simulink model "geometric_control"  (R2023b)
settings: Solver=VariableStepAuto  StartTime=0.0  StopTime=20.0  RelTol=1e-3
InitFcn:
  | %% INITFNC - Ground Effect
  | %% UAV PARAMETERS
  | mass = 4.34;
  | Ib = diag([0.08, 0.08, 0.14]);
  | rho = 0.05;
  | d = 0.42;
  | 
  | %% SAMPLING TIME
  | Ts = 0.001;
  | 
  | %% TRAJECTORY SETTINGS
  | t_iniz = 0;
  | tdead=10;
  | tot_time = 20;
  | t = linspace(0, tot_time, round(tot_time/Ts));
  | 
  | 
  | z_d = zeros(size(t));
  | dz_d = zeros(size(t));
  | ddz_d = zeros(size(t));
  | 
  | for i = 1:length(t)
  |     ti = t(i);
  |     if ti < 2.5
  |         z_d(i) = 0.05 + (1.5 - 0.05) / 2.5 * ti;
  |         dz_d(i) = (1.5 - 0.05) / 2.5;
  |         ddz_d(i) = 0;
  |     elseif ti < 5
  |         z_d(i) = 1.5;
  |         dz_d(i) = 0;
  |         ddz_d(i) = 0;
  |     elseif ti < 7.5
  |         z_d(i) = 1.5 - (1.5 - 0.1) / 2.5 * (ti - 5);
  |         dz_d(i) = -(1.5 - 0.1) / 2.5;
  |         ddz_d(i) = 0;
  |     else
  |         z_d(i) = 0.1;
  |         dz_d(i) = 0;
  |         ddz_d(i) = 0;
  |     end
  | end
  | 
  | 
  | x_d = zeros(size(t));
  | y_d = zeros(size(t));
  | psi_d = zeros(size(t));
  | 
  | dx_d = zeros(size(t));
  | dy_d = zeros(size(t));
  | dot_psi_d = zeros(size(t));
  | 
  | ddx_d = zeros(size(t));
  | ddy_d = zeros(size(t));
  | ddot_psi_d = zeros(size(t));
  | 
  | p_d = [x_d; y_d; z_d; psi_d];
  | dot_p_d = [dx_d; dy_d; dz_d; dot_psi_d];
  | ddot_p_d = [ddx_d; ddy_d; ddz_d; ddot_psi_d];
  | 
  | p_final = p_d(:, end);
  | dot_p_final = dot_p_d(:, end);
  | ddot_p_final = ddot_p_d(:, end);
  | 
  | n_dead = round(tdead / Ts);
  | p_d = [p_d, repmat(p_final, 1, n_dead)];
  | dot_p_d = [dot_p_d, repmat(dot_p_final, 1, n_dead)];
  | ddot_p_d = [ddot_p_d, repmat(ddot_p_final, 1, n_dead)];
  | 
  | target_len = length(t);
  | p_d = p_d(:, 1:target_len);
  | dot_p_d = dot_p_d(:, 1:target_len);
  | ddot_p_d = ddot_p_d(:, 1:target_len);
  | 
  | %% OUTPUTS FOR SIMULINK
  | x0 = p_d(1,1); y0 = p_d(2,1); z0 = p_d(3,1);
  | pos_0 = [x0 y0 z0];
  | lin_vel_0 = [dot_p_d(1,1), dot_p_d(2,1), dot_p_d(3,1)];
  | w_bb_0 = [0 0 0];
  | 
  | csi_d = p_d(1:3,:);
  | dot_csi_d = dot_p_d(1:3,:);
  | ddot_csi_d = ddot_p_d(1:3,:);
  | 
  | psi_d = p_d(4,:);
  | dot_psi_d = dot_p_d(4,:);
  | ddot_psi_d = ddot_p_d(4,:);
libraries: robotcorelib x2, uavutilslib x2
settings Model: Creator=fabioruggiero  LastModifiedBy=lidia
settings ModelReferenceCC: EnableRefExpFcnMdlSchedulingChecks=on

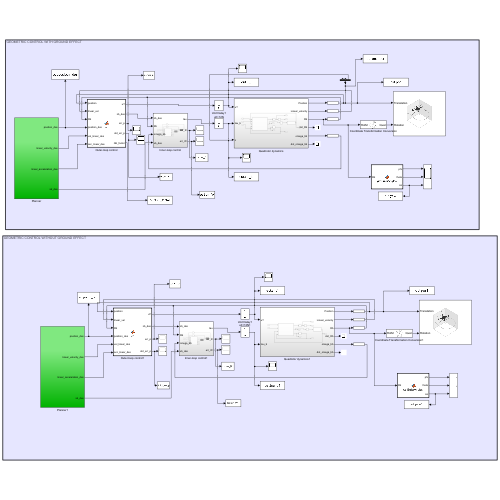
[thumbnail: Simulink's stored preview of the top-level diagram]
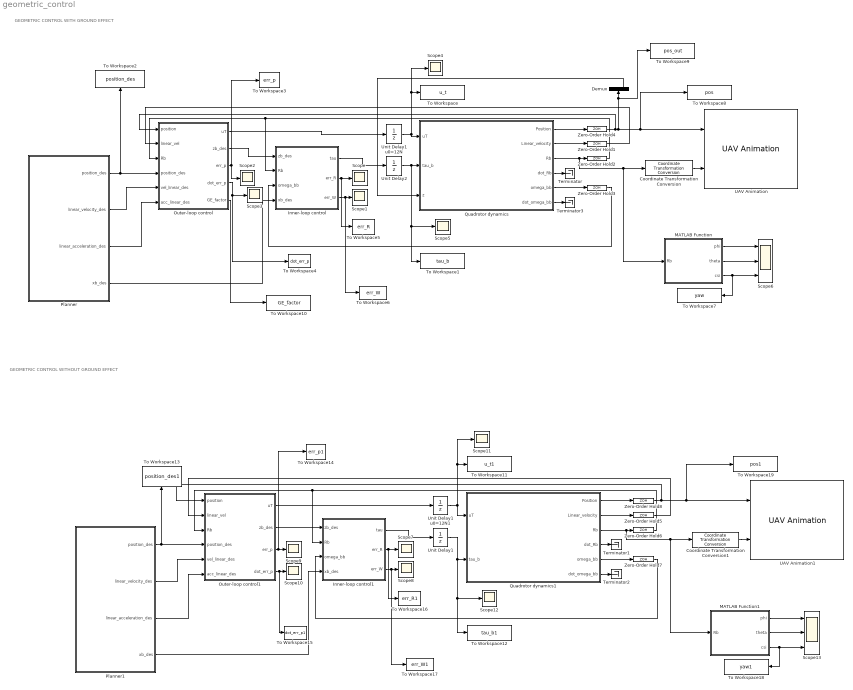
== system geometric_control ==
  note: GEOMETRIC CONTROL WITHOUT GROUND EFFECT
  note: GEOMETRIC CONTROL WITH GROUND EFFECT
  Coordinate Transformation Conversion : robotcorelib/Coordinate Transformation Conversion  InputRepresentation=Rotation Matrix  InputEulerSequence=ZYX  ShowTrVecInputPort=on  OutputRepresentation=Quaternion  OutputEulerSequence=ZYX  ShowTrVecOutputPort=on  SimulateUsing=Interpreted execution
  Coordinate Transformation Conversion1 : robotcorelib/Coordinate Transformation Conversion  InputRepresentation=Rotation Matrix  InputEulerSequence=ZYX  ShowTrVecInputPort=on  OutputRepresentation=Quaternion  OutputEulerSequence=ZYX  ShowTrVecOutputPort=on  SimulateUsing=Interpreted execution
  Demux : Demux  Outputs=3
  Inner-loop control : Subsystem
  Inner-loop control1 : Subsystem
  MATLAB Function : MATLAB Function  TreatAsAtomicUnit=on
  MATLAB Function1 : MATLAB Function  TreatAsAtomicUnit=on
  Outer-loop control : MATLAB Function  TreatAsAtomicUnit=on
  Outer-loop control1 : MATLAB Function  TreatAsAtomicUnit=on
  Planner : Subsystem
  Planner1 : Subsystem
  Quadrotor dynamics : Subsystem
  Quadrotor dynamics1 : Subsystem
  Scope{,1..5,7..12} (12 alike) : Scope
  Scope13 : Scope  NumInputPorts=3
  Scope6 : Scope  NumInputPorts=3
  Terminator{,1..3} (4 alike) : Terminator
  To Workspace : ToWorkspace  VariableName=u_t  SaveFormat=Timeseries  SampleTime=-1
  To Workspace1 : ToWorkspace  VariableName=tau_b  SaveFormat=Timeseries  SampleTime=-1
  To Workspace10 : ToWorkspace  VariableName=GE_factor  SaveFormat=Timeseries  SampleTime=-1
  To Workspace11 : ToWorkspace  VariableName=u_t1  SaveFormat=Timeseries  SampleTime=-1
  To Workspace12 : ToWorkspace  VariableName=tau_b1  SaveFormat=Timeseries  SampleTime=-1
  To Workspace13 : ToWorkspace  VariableName=position_des1  SaveFormat=Timeseries  SampleTime=-1
  To Workspace14 : ToWorkspace  VariableName=err_p1  SaveFormat=Timeseries  SampleTime=-1
  To Workspace15 : ToWorkspace  VariableName=dot_err_p1  SaveFormat=Timeseries  SampleTime=-1
  To Workspace16 : ToWorkspace  VariableName=err_R1  SaveFormat=Timeseries  SampleTime=-1
  To Workspace17 : ToWorkspace  VariableName=err_W1  SaveFormat=Timeseries  SampleTime=-1
  To Workspace18 : ToWorkspace  VariableName=yaw1  SaveFormat=Timeseries  SampleTime=-1
  To Workspace19 : ToWorkspace  VariableName=pos1  SaveFormat=Timeseries  SampleTime=-1
  To Workspace2 : ToWorkspace  VariableName=position_des  SaveFormat=Timeseries  SampleTime=-1
  To Workspace3 : ToWorkspace  VariableName=err_p  SaveFormat=Timeseries  SampleTime=-1
  To Workspace4 : ToWorkspace  VariableName=dot_err_p  SaveFormat=Timeseries  SampleTime=-1
  To Workspace5 : ToWorkspace  VariableName=err_R  SaveFormat=Timeseries  SampleTime=-1
  To Workspace6 : ToWorkspace  VariableName=err_W  SaveFormat=Timeseries  SampleTime=-1
  To Workspace7 : ToWorkspace  VariableName=yaw  SaveFormat=Timeseries  SampleTime=-1
  To Workspace8 : ToWorkspace  VariableName=pos  SaveFormat=Timeseries  SampleTime=-1
  To Workspace9 : ToWorkspace  VariableName=pos_out  SaveFormat=Structure With Time  SampleTime=Ts
  UAV Animation : uavutilslib/UAV Animation  UAVType=Multirotor  UAVSize=1  InertialZDirection=Down  SampleTime=0.01
  UAV Animation1 : uavutilslib/UAV Animation  UAVType=Multirotor  UAVSize=1  InertialZDirection=Down  SampleTime=0.01
  Unit Delay1 : UnitDelay  InitialCondition=[0 0 0]  SampleTime=Ts
  Unit Delay1 u0=12N : UnitDelay  InitialCondition=12  SampleTime=Ts
  Unit Delay1 u0=12N1 : UnitDelay  InitialCondition=12  SampleTime=Ts
  Unit Delay2 : UnitDelay  InitialCondition=[0 0 0]  SampleTime=Ts
  Zero-Order Hold{1..8} (8 alike) : ZeroOrderHold  SampleTime=Ts
  wires:
  Outer-loop control/1(uT) -> Unit Delay1 u0=12N/1
  Unit Delay1 u0=12N/1 -> Quadrotor dynamics/1(uT), To Workspace/1, Scope4/1
  Quadrotor dynamics/1(Position) -> Zero-Order Hold4/1
  Quadrotor dynamics/2(Linear_velocity) -> Zero-Order Hold1/1
  Quadrotor dynamics/3(Rb) -> Coordinate Transformation Conversion/1, MATLAB Function/1(Rb), Zero-Order Hold2/1
  Quadrotor dynamics/5(omega_bb) -> Zero-Order Hold3/1
  Zero-Order Hold4/1 -> To Workspace9/1, Demux/1, To Workspace8/1, UAV Animation/1, Outer-loop control/1(position)
  Zero-Order Hold1/1 -> Outer-loop control/2(linear_vel)
  Zero-Order Hold2/1 -> Outer-loop control/3(Rb), Inner-loop control/2(Rb)
  Unit Delay2/1 -> To Workspace1/1, Scope5/1, Quadrotor dynamics/2(tau_b)
  Quadrotor dynamics/4(dot_Rb) -> Terminator/1
  Planner/1(position_des) -> To Workspace2/1, Outer-loop control/4(position_des)
  Planner/2(linear_velocity_des) -> Outer-loop control/5(vel_linear_des)
  Planner/3(linear_acceleration_des) -> Outer-loop control/6(acc_linear_des)
  Planner/4(xb_des) -> Inner-loop control/4(xb_des)
  Outer-loop control/3(err_p) -> Scope2/1, To Workspace3/1
  Outer-loop control/4(dot_err_p) -> To Workspace4/1, Scope3/1
  Quadrotor dynamics/6(dot_omega_bb) -> Terminator3/1
  Coordinate Transformation Conversion/1 -> UAV Animation/2
  Outer-loop control/2(zb_des) -> Inner-loop control/1(zb_des)
  Zero-Order Hold3/1 -> Inner-loop control/3(omega_bb)
  Inner-loop control/1(tau) -> Unit Delay2/1
  Inner-loop control/2(err_R) -> To Workspace5/1, Scope/1
  Inner-loop control/3(err_W) -> To Workspace6/1, Scope1/1
  MATLAB Function/1(phi) -> Scope6/1
  MATLAB Function/2(theta) -> Scope6/2
  MATLAB Function/3(csi) -> To Workspace7/1, Scope6/3
  Demux/3 -> Quadrotor dynamics/3(z)
  Outer-loop control/5(GE_factor) -> To Workspace10/1
  Planner1/3(linear_acceleration_des) -> Outer-loop control1/6(acc_linear_des)
  MATLAB Function1/1(phi) -> Scope13/1
  Outer-loop control1/3(err_p) -> To Workspace14/1, Scope9/1
  MATLAB Function1/3(csi) -> To Workspace18/1, Scope13/3
  Zero-Order Hold7/1 -> Inner-loop control1/3(omega_bb)
  MATLAB Function1/2(theta) -> Scope13/2
  Inner-loop control1/1(tau) -> Unit Delay1/1
  Quadrotor dynamics1/2(Linear_velocity) -> Zero-Order Hold5/1
  Inner-loop control1/3(err_W) -> To Workspace17/1, Scope8/1
  Planner1/4(xb_des) -> Inner-loop control1/4(xb_des)
  Quadrotor dynamics1/6(dot_omega_bb) -> Terminator2/1
  Zero-Order Hold8/1 -> To Workspace19/1, UAV Animation1/1, Outer-loop control1/1(position)
  Quadrotor dynamics1/4(dot_Rb) -> Terminator1/1
  Planner1/2(linear_velocity_des) -> Outer-loop control1/5(vel_linear_des)
  Planner1/1(position_des) -> Outer-loop control1/4(position_des), To Workspace13/1
  Outer-loop control1/4(dot_err_p) -> To Workspace15/1, Scope10/1
  Quadrotor dynamics1/3(Rb) -> Coordinate Transformation Conversion1/1, MATLAB Function1/1(Rb), Zero-Order Hold6/1
  Coordinate Transformation Conversion1/1 -> UAV Animation1/2
  Outer-loop control1/2(zb_des) -> Inner-loop control1/1(zb_des)
  Quadrotor dynamics1/5(omega_bb) -> Zero-Order Hold7/1
  Zero-Order Hold5/1 -> Outer-loop control1/2(linear_vel)
  Inner-loop control1/2(err_R) -> To Workspace16/1, Scope7/1
  Unit Delay1/1 -> To Workspace12/1, Scope12/1, Quadrotor dynamics1/2(tau_b)
  Outer-loop control1/1(uT) -> Unit Delay1 u0=12N1/1
  Zero-Order Hold6/1 -> Outer-loop control1/3(Rb), Inner-loop control1/2(Rb)
  Unit Delay1 u0=12N1/1 -> Quadrotor dynamics1/1(uT), To Workspace11/1, Scope11/1
  Quadrotor dynamics1/1(Position) -> Zero-Order Hold8/1

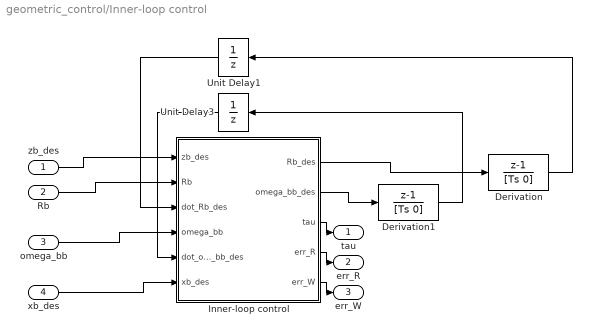
== system geometric_control/Inner-loop control ==
  zb_des : Inport
  Rb : Inport  Port=2
  omega_bb : Inport  Port=3
  xb_des : Inport  Port=4
  Derivation : DiscreteTransferFcn  Numerator=[1 -1]  Denominator=[Ts 0]  InitialStates=[1 0 0;0 1 0;0 0 1]  SampleTime=Ts
  Derivation1 : DiscreteTransferFcn  Numerator=[1 -1]  Denominator=[Ts 0]  InitialStates=[0 0 0]  SampleTime=Ts
  Inner-loop control : MATLAB Function  TreatAsAtomicUnit=on
  Unit Delay1 : UnitDelay  InitialCondition=eye(3)  SampleTime=Ts
  Unit Delay3 : UnitDelay  InitialCondition=[0 0 0]  SampleTime=Ts
  tau : Outport
  err_R : Outport  Port=2
  err_W : Outport  Port=3
  wires:
  xb_des/1 -> Inner-loop control/6(xb_des)
  Inner-loop control/4(err_R) -> err_R/1
  Rb/1 -> Inner-loop control/2(Rb)
  Inner-loop control/3(tau) -> tau/1
  Unit Delay1/1 -> Inner-loop control/3(dot_Rb_des)
  Derivation1/1 -> Unit Delay3/1
  Inner-loop control/5(err_W) -> err_W/1
  Unit Delay3/1 -> Inner-loop control/5(dot_omega_bb_des)
  Derivation/1 -> Unit Delay1/1
  zb_des/1 -> Inner-loop control/1(zb_des)
  omega_bb/1 -> Inner-loop control/4(omega_bb)
  Inner-loop control/1(Rb_des) -> Derivation/1
  Inner-loop control/2(omega_bb_des) -> Derivation1/1

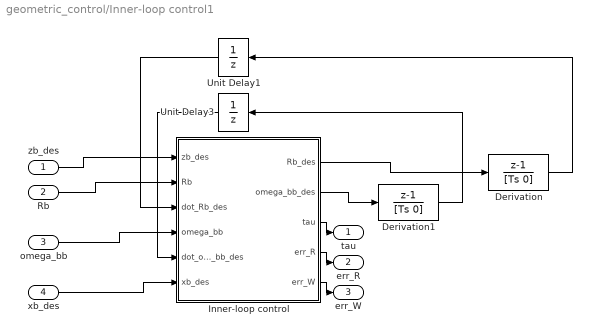
== system geometric_control/Inner-loop control1 ==
  zb_des : Inport
  Rb : Inport  Port=2
  omega_bb : Inport  Port=3
  xb_des : Inport  Port=4
  Derivation : DiscreteTransferFcn  Numerator=[1 -1]  Denominator=[Ts 0]  InitialStates=[1 0 0;0 1 0;0 0 1]  SampleTime=Ts
  Derivation1 : DiscreteTransferFcn  Numerator=[1 -1]  Denominator=[Ts 0]  InitialStates=[0 0 0]  SampleTime=Ts
  Inner-loop control : MATLAB Function  TreatAsAtomicUnit=on
  Unit Delay1 : UnitDelay  InitialCondition=eye(3)  SampleTime=Ts
  Unit Delay3 : UnitDelay  InitialCondition=[0 0 0]  SampleTime=Ts
  tau : Outport
  err_R : Outport  Port=2
  err_W : Outport  Port=3
  wires:
  xb_des/1 -> Inner-loop control/6(xb_des)
  Inner-loop control/4(err_R) -> err_R/1
  Rb/1 -> Inner-loop control/2(Rb)
  Inner-loop control/3(tau) -> tau/1
  Unit Delay1/1 -> Inner-loop control/3(dot_Rb_des)
  Derivation1/1 -> Unit Delay3/1
  Inner-loop control/5(err_W) -> err_W/1
  Unit Delay3/1 -> Inner-loop control/5(dot_omega_bb_des)
  Derivation/1 -> Unit Delay1/1
  zb_des/1 -> Inner-loop control/1(zb_des)
  omega_bb/1 -> Inner-loop control/4(omega_bb)
  Inner-loop control/1(Rb_des) -> Derivation/1
  Inner-loop control/2(omega_bb_des) -> Derivation1/1

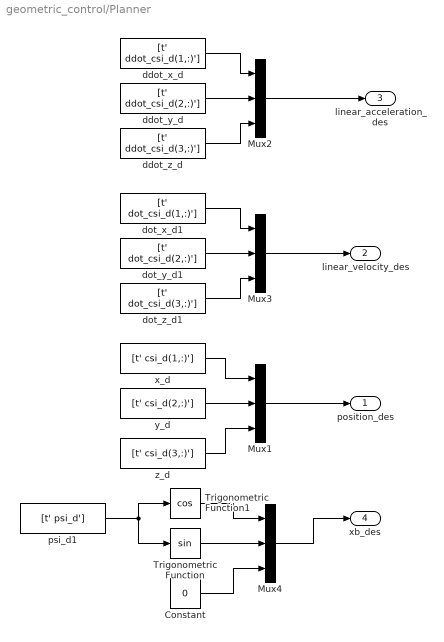
== system geometric_control/Planner ==
  Constant : Constant  Value=0
  Mux{1..4} (4 alike) : Mux  Inputs=3
  Trigonometric Function : Trigonometry
  Trigonometric Function1 : Trigonometry  Operator=cos
  ddot_x_d : FromWorkspace  VariableName=[t' ddot_csi_d(1,:)']  SampleTime=Ts
  ddot_y_d : FromWorkspace  VariableName=[t' ddot_csi_d(2,:)']  SampleTime=Ts
  ddot_z_d : FromWorkspace  VariableName=[t' ddot_csi_d(3,:)']  SampleTime=Ts
  dot_x_d1 : FromWorkspace  VariableName=[t' dot_csi_d(1,:)']  SampleTime=Ts
  dot_y_d1 : FromWorkspace  VariableName=[t' dot_csi_d(2,:)']  SampleTime=Ts
  dot_z_d1 : FromWorkspace  VariableName=[t' dot_csi_d(3,:)']  SampleTime=Ts
  psi_d1 : FromWorkspace  VariableName=[t' psi_d']  SampleTime=Ts
  x_d : FromWorkspace  VariableName=[t' csi_d(1,:)']  SampleTime=Ts
  y_d : FromWorkspace  VariableName=[t' csi_d(2,:)']  SampleTime=Ts
  z_d : FromWorkspace  VariableName=[t' csi_d(3,:)']  SampleTime=Ts
  position_des : Outport
  linear_velocity_des : Outport  Port=2
  linear_acceleration_des : Outport  Port=3
  xb_des : Outport  Port=4
  wires:
  y_d/1 -> Mux1/2
  z_d/1 -> Mux1/3
  x_d/1 -> Mux1/1
  ddot_y_d/1 -> Mux2/2
  ddot_z_d/1 -> Mux2/3
  ddot_x_d/1 -> Mux2/1
  Mux2/1 -> linear_acceleration_des/1
  Mux1/1 -> position_des/1
  dot_y_d1/1 -> Mux3/2
  dot_z_d1/1 -> Mux3/3
  dot_x_d1/1 -> Mux3/1
  Mux3/1 -> linear_velocity_des/1
  Mux4/1 -> xb_des/1
  Trigonometric Function/1 -> Mux4/2
  psi_d1/1 -> Trigonometric Function/1, Trigonometric Function1/1
  Trigonometric Function1/1 -> Mux4/1
  Constant/1 -> Mux4/3

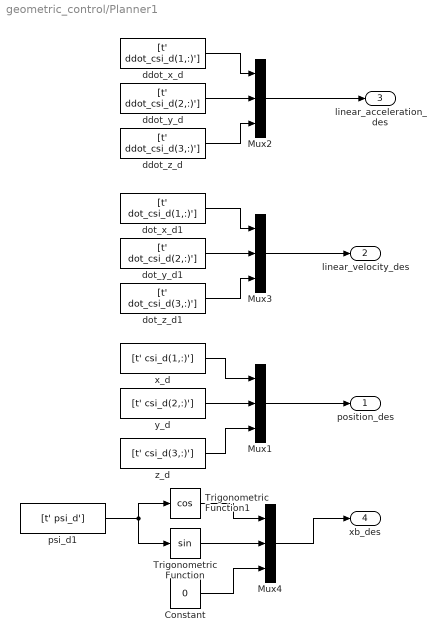
== system geometric_control/Planner1 ==
  Constant : Constant  Value=0
  Mux{1..4} (4 alike) : Mux  Inputs=3
  Trigonometric Function : Trigonometry
  Trigonometric Function1 : Trigonometry  Operator=cos
  ddot_x_d : FromWorkspace  VariableName=[t' ddot_csi_d(1,:)']  SampleTime=Ts
  ddot_y_d : FromWorkspace  VariableName=[t' ddot_csi_d(2,:)']  SampleTime=Ts
  ddot_z_d : FromWorkspace  VariableName=[t' ddot_csi_d(3,:)']  SampleTime=Ts
  dot_x_d1 : FromWorkspace  VariableName=[t' dot_csi_d(1,:)']  SampleTime=Ts
  dot_y_d1 : FromWorkspace  VariableName=[t' dot_csi_d(2,:)']  SampleTime=Ts
  dot_z_d1 : FromWorkspace  VariableName=[t' dot_csi_d(3,:)']  SampleTime=Ts
  psi_d1 : FromWorkspace  VariableName=[t' psi_d']  SampleTime=Ts
  x_d : FromWorkspace  VariableName=[t' csi_d(1,:)']  SampleTime=Ts
  y_d : FromWorkspace  VariableName=[t' csi_d(2,:)']  SampleTime=Ts
  z_d : FromWorkspace  VariableName=[t' csi_d(3,:)']  SampleTime=Ts
  position_des : Outport
  linear_velocity_des : Outport  Port=2
  linear_acceleration_des : Outport  Port=3
  xb_des : Outport  Port=4
  wires:
  y_d/1 -> Mux1/2
  z_d/1 -> Mux1/3
  x_d/1 -> Mux1/1
  ddot_y_d/1 -> Mux2/2
  ddot_z_d/1 -> Mux2/3
  ddot_x_d/1 -> Mux2/1
  Mux2/1 -> linear_acceleration_des/1
  Mux1/1 -> position_des/1
  dot_y_d1/1 -> Mux3/2
  dot_z_d1/1 -> Mux3/3
  dot_x_d1/1 -> Mux3/1
  Mux3/1 -> linear_velocity_des/1
  Mux4/1 -> xb_des/1
  Trigonometric Function/1 -> Mux4/2
  psi_d1/1 -> Trigonometric Function/1, Trigonometric Function1/1
  Trigonometric Function1/1 -> Mux4/1
  Constant/1 -> Mux4/3

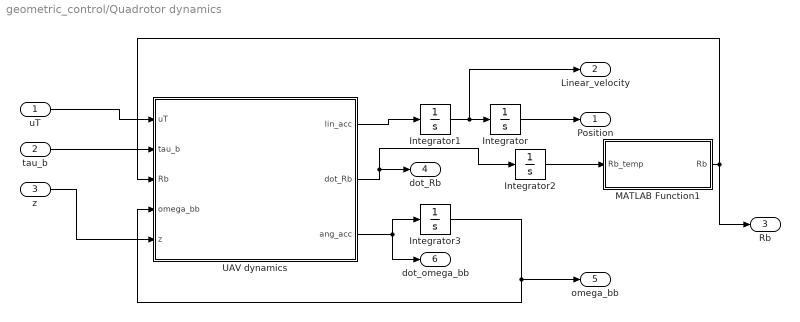
== system geometric_control/Quadrotor dynamics ==
  uT : Inport
  tau_b : Inport  Port=2
  z : Inport  Port=3
  Integrator : Integrator  InitialCondition=pos_0
  Integrator1 : Integrator  InitialCondition=lin_vel_0
  Integrator2 : Integrator  InitialCondition=[1 0 0; 0 1 0;0 0 1]
  Integrator3 : Integrator  InitialCondition=w_bb_0
  MATLAB Function1 : MATLAB Function  TreatAsAtomicUnit=on
  UAV dynamics : MATLAB Function  TreatAsAtomicUnit=on
  Position : Outport
  Linear_velocity : Outport  Port=2
  Rb : Outport  Port=3
  dot_Rb : Outport  Port=4
  omega_bb : Outport  Port=5
  dot_omega_bb : Outport  Port=6
  wires:
  tau_b/1 -> UAV dynamics/2(tau_b)
  Integrator/1 -> Position/1
  UAV dynamics/3(ang_acc) -> Integrator3/1, dot_omega_bb/1
  UAV dynamics/1(lin_acc) -> Integrator1/1
  uT/1 -> UAV dynamics/1(uT)
  Integrator1/1 -> Linear_velocity/1, Integrator/1
  Integrator3/1 -> UAV dynamics/4(omega_bb), omega_bb/1
  UAV dynamics/2(dot_Rb) -> Integrator2/1, dot_Rb/1
  MATLAB Function1/1(Rb) -> Rb/1, UAV dynamics/3(Rb)
  Integrator2/1 -> MATLAB Function1/1(Rb_temp)
  z/1 -> UAV dynamics/5(z)

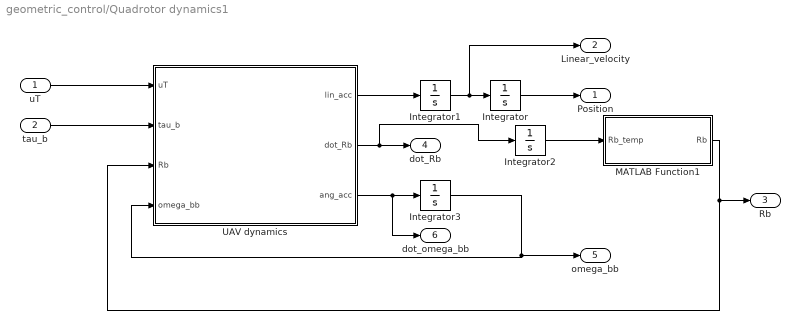
== system geometric_control/Quadrotor dynamics1 ==
  uT : Inport
  tau_b : Inport  Port=2
  Integrator : Integrator  InitialCondition=pos_0
  Integrator1 : Integrator  InitialCondition=lin_vel_0
  Integrator2 : Integrator  InitialCondition=[1 0 0; 0 1 0;0 0 1]
  Integrator3 : Integrator  InitialCondition=w_bb_0
  MATLAB Function1 : MATLAB Function  TreatAsAtomicUnit=on
  UAV dynamics : MATLAB Function  TreatAsAtomicUnit=on
  Position : Outport
  Linear_velocity : Outport  Port=2
  Rb : Outport  Port=3
  dot_Rb : Outport  Port=4
  omega_bb : Outport  Port=5
  dot_omega_bb : Outport  Port=6
  wires:
  tau_b/1 -> UAV dynamics/2(tau_b)
  Integrator/1 -> Position/1
  UAV dynamics/3(ang_acc) -> dot_omega_bb/1, Integrator3/1
  UAV dynamics/1(lin_acc) -> Integrator1/1
  uT/1 -> UAV dynamics/1(uT)
  Integrator1/1 -> Linear_velocity/1, Integrator/1
  Integrator3/1 -> UAV dynamics/4(omega_bb), omega_bb/1
  UAV dynamics/2(dot_Rb) -> Integrator2/1, dot_Rb/1
  MATLAB Function1/1(Rb) -> Rb/1, UAV dynamics/3(Rb)
  Integrator2/1 -> MATLAB Function1/1(Rb_temp)

== matlab function geometric_control/MATLAB Function1 ==
  data: Rb input; phi output; theta output; csi output
function [phi, theta, csi] = getEulerAngles(Rb)

    phi   = rad2deg(atan2(Rb(3,2), Rb(3,3)));    % roll
    theta = rad2deg(-asin(Rb(3,1)));             % pitch
    csi   = rad2deg(atan2(Rb(2,1), Rb(1,1)));    % yaw
    
end

== matlab function geometric_control/Outer-loop control1 ==
  data: position input size=3; uT output size=1; linear_vel input size=3; Rb input size=[3,3]; zb_des output size=3; mass parameter size=1; position_des input size=3; vel_linear_des input size=3; acc_linear_des input size=3; err_p output size=3; dot_err_p output size=3
function [uT, zb_des, err_p, dot_err_p] = fcn(position, linear_vel, Rb, mass, ...
    position_des, vel_linear_des, acc_linear_des)

g=9.81;
e_3=[0 0 1]';
Kp=diag([13,13,13]);
Kv=diag([8,8,8]);
err_p=position-position_des;
dot_err_p= linear_vel-vel_linear_des;
uT=-[(-Kp*err_p-Kv*dot_err_p-mass*g*e_3+mass*acc_linear_des)']*Rb*e_3;
zb_des=-[-Kp*err_p-Kv*dot_err_p-mass*g*e_3+mass*acc_linear_des]/norm(-Kp*err_p-Kv*dot_err_p-mass*g*e_3+mass*acc_linear_des);

== matlab function geometric_control/Quadrotor dynamics1/MATLAB Function1 ==
  data: Rb_temp input; Rb output
function Rb = fcn(Rb_temp)
    [U,S,V] = svd(Rb_temp);
    sigma = det(U*V');
    S_ = diag([1 1 sigma]);

    Rb = U*S_*V';
end

== matlab function geometric_control/Quadrotor dynamics1/UAV dynamics ==
  data: uT input size=1; tau_b input size=3; lin_acc output size=3; Rb input size=[3,3]; omega_bb input size=3; dot_Rb output size=[3,3]; ang_acc output size=3; mass parameter size=1; Ib parameter size=[3,3]
function [lin_acc, dot_Rb, ang_acc] = fcn(uT,tau_b,Rb,omega_bb,mass, Ib)

lin_acc = 9.81*[0 0 1]'-(uT/mass)*Rb*[0 0 1]';
dot_Rb = Rb*skew(omega_bb);
ang_acc = inv(Ib)*(-skew(omega_bb)*Ib*omega_bb + tau_b);

end

function S = skew(v)
if(numel(v)~= 1)
S= [0 -v(3) v(2); 
    v(3) 0 -v(1);
    -v(2) v(1) 0];
else
S= zeros(3);
end
end

== matlab function geometric_control/MATLAB Function ==
  data: Rb input; phi output; theta output; csi output
function [phi, theta, csi] = getEulerAngles(Rb)

    phi   = rad2deg(atan2(Rb(3,2), Rb(3,3)));    % roll
    theta = rad2deg(-asin(Rb(3,1)));             % pitch
    csi   = rad2deg(atan2(Rb(2,1), Rb(1,1)));    % yaw
    
end

== matlab function geometric_control/Quadrotor dynamics/UAV dynamics ==
  data: uT input size=1; tau_b input size=3; lin_acc output size=3; Rb input size=[3,3]; omega_bb input size=3; dot_Rb output size=[3,3]; ang_acc output size=3; mass parameter size=1; Ib parameter size=[3,3]; z input; rho parameter; d parameter
function [lin_acc, dot_Rb, ang_acc] = fcn(uT,tau_b,Rb,omega_bb,mass, Ib, z, rho, d)
 

if z > 2*rho
    GE_factor = 1; 
else
    Z = 1; 
    term1 = (rho^2)/(4*z^2);
    term2 = Z * rho^2 / ((d^2 + 4*z^2)^(3/2));
    term3 = Z * rho^2 / ((2*d^2 + 4*z^2)^(3/2));
    GE_factor = 1 / (1 - term1 - term2 - term3);
end
 

uT_corr = GE_factor * uT;
 

lin_acc = 9.81*[0 0 1]' - (uT_corr/mass)*Rb*[0 0 1]';
 

dot_Rb = Rb * skew(omega_bb);
 

ang_acc = inv(Ib)*(-skew(omega_bb)*Ib*omega_bb + tau_b);
 
end
 
function S = skew(v)
if(numel(v)~= 1)
S= [0 -v(3) v(2); 
    v(3) 0 -v(1);
    -v(2) v(1) 0];
else
S= zeros(3);
end
end

== matlab function geometric_control/Outer-loop control ==
  data: position input size=3; uT output size=1; linear_vel input size=3; Rb input size=[3,3]; zb_des output size=3; mass parameter size=1; position_des input size=3; vel_linear_des input size=3; acc_linear_des input size=3; err_p output size=3; dot_err_p output size=3; rho parameter; d parameter; GE_factor output
function [uT, zb_des, err_p, dot_err_p,GE_factor] = fcn(position, linear_vel, Rb, mass, ...
    position_des, vel_linear_des, acc_linear_des, rho, d)


g = 9.81;
e_3 = [0 0 1]';
Kp = diag([13, 13, 13]);
Kv = diag([8, 8, 8]);

err_p = position - position_des;
dot_err_p = linear_vel - vel_linear_des;

F = -Kp * err_p - Kv * dot_err_p - mass * g * e_3 + mass * acc_linear_des;

%% GROUND EFFECT CORRECTION
z = max(position(3), 0.05); 
if z > 2 * rho
    GE_factor = 1;
else
    Z = 1;  
    term1 = (rho^2) / (4 * z^2);
    term2 = Z * rho^2 / ((d^2 + 4 * z^2)^(3/2));
    term3 = Z * rho^2 / ((2 * d^2 + 4 * z^2)^(3/2));
    denom = 1 - term1 - term2 - term3;

    if denom < 0.05 
        GE_factor = 1;
    else
        GE_factor = 1 / denom;
    end
end


uT = -F' * Rb * e_3 / GE_factor;


zb_des = -F / norm(F);
end

== matlab function geometric_control/Inner-loop control/Inner-loop control ==
  data: Rb_des output size=[3,3]; omega_bb_des output size=3; tau output size=3; zb_des input size=3; Rb input size=[3,3]; dot_Rb_des input size=[3,3]; omega_bb input size=3; dot_omega_bb_des input size=3; xb_des input size=3; Ib parameter size=[3,3]; err_R output size=3; err_W output size=3
function [Rb_des,omega_bb_des,tau,err_R,err_W] = fcn(zb_des,Rb,dot_Rb_des,omega_bb,dot_omega_bb_des,xb_des,Ib)


yb_des = cross(zb_des, xb_des) / norm(cross(zb_des, xb_des));
Rb_des=[skew(yb_des)*zb_des, yb_des, zb_des];
err_R=0.5*wedge((Rb_des'*Rb-Rb'*Rb_des));
omega_bb_des = wedge(Rb_des'*dot_Rb_des);
err_W=omega_bb-Rb'*Rb_des*omega_bb_des;
Kr=diag([30,30,30]);
Kw=diag([5,5,5]);
tau=-Kr*err_R-Kw*err_W+skew(omega_bb)*Ib*omega_bb-Ib*(skew(omega_bb)*Rb'*Rb_des*omega_bb_des-Rb'*Rb_des*dot_omega_bb_des);
end

function S = skew(v)
if(numel(v)~= 1)
S= [0 -v(3) v(2); 
    v(3) 0 -v(1);
    -v(2) v(1) 0];
else
S= zeros(3);
end
end

function v = wedge(S)
v1 = S(3,2);
v2 = S(1,3);
v3 = S(2,1);
v = [v1 v2 v3]';
end

== matlab function geometric_control/Quadrotor dynamics/MATLAB Function1 ==
  data: Rb_temp input; Rb output
function Rb = fcn(Rb_temp)
    [U,S,V] = svd(Rb_temp);
    sigma = det(U*V');
    S_ = diag([1 1 sigma]);

    Rb = U*S_*V';
end

== matlab function geometric_control/Inner-loop control1/Inner-loop control ==
  data: Rb_des output size=[3,3]; omega_bb_des output size=3; tau output size=3; zb_des input size=3; Rb input size=[3,3]; dot_Rb_des input size=[3,3]; omega_bb input size=3; dot_omega_bb_des input size=3; xb_des input size=3; Ib parameter size=[3,3]; err_R output size=3; err_W output size=3
function [Rb_des,omega_bb_des,tau,err_R,err_W] = fcn(zb_des,Rb,dot_Rb_des,omega_bb,dot_omega_bb_des,xb_des,Ib)


yb_des = cross(zb_des, xb_des) / norm(cross(zb_des, xb_des));
Rb_des=[skew(yb_des)*zb_des, yb_des, zb_des];
err_R=0.5*wedge((Rb_des'*Rb-Rb'*Rb_des));
omega_bb_des = wedge(Rb_des'*dot_Rb_des);
err_W=omega_bb-Rb'*Rb_des*omega_bb_des;
Kr=diag([30,30,30]);
Kw=diag([5,5,5]);
tau=-Kr*err_R-Kw*err_W+skew(omega_bb)*Ib*omega_bb-Ib*(skew(omega_bb)*Rb'*Rb_des*omega_bb_des-Rb'*Rb_des*dot_omega_bb_des);
end

function S = skew(v)
if(numel(v)~= 1)
S= [0 -v(3) v(2); 
    v(3) 0 -v(1);
    -v(2) v(1) 0];
else
S= zeros(3);
end
end

function v = wedge(S)
v1 = S(3,2);
v2 = S(1,3);
v3 = S(2,1);
v = [v1 v2 v3]';
end
